simulink model "Problem1"  (R2020b)
settings: Solver=VariableStepAuto  StartTime=0.0  StopTime=120  RelTol=1e-3
model workspace (MAT data in the model file):
  b = Simulink.Parameter
  b.Value = 50
  b.DataType = 'auto'
  b.Dimensions = [1 1]
  m = Simulink.Parameter
  m.Value = 1000
  m.DataType = 'auto'
  m.Dimensions = [1 1]
  u = Simulink.Parameter
  u.Value = 500
  u.DataType = 'auto'
  u.Dimensions = [1 1]
settings Model: Creator=Hp  LastModifiedBy=Hp

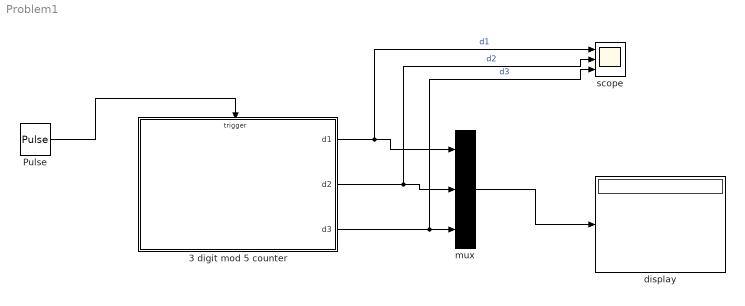
== system Problem1 ==
  3 digit mod 5 counter : Stateflow chart  TreatAsAtomicUnit=on
  Pulse : DiscretePulseGenerator  PulseType=Time based  Period=1  PulseWidth=5
  display : Display
  mux : Mux  Inputs=3
  scope : Scope  NumInputPorts=3
  wires:
  Pulse/1 -> 3 digit mod 5 counter/Trigger
  mux/1 -> display/1
  3 digit mod 5 counter/3(d3) -> scope/3, mux/3  "d3"
  3 digit mod 5 counter/2(d2) -> scope/2, mux/2  "d2"
  3 digit mod 5 counter/1(d1) -> scope/1, mux/1  "d1"

== stateflow chart Problem1/3 digit mod 5 counter ==
  state digit1 [parallel]
    settings: executionOrder=1
    state zero
      en:d1=0;
    state four
      en:d1=4;
    state one
      en:d1=1;
    state three
      en:d1=3;
    state two
      en:d1=2;
    (default) -> digit1.zero
    digit1.zero -> digit1.one : inputClick
    digit1.four -> digit1.zero : inputClick/{digit2.inc2}
    digit1.three -> digit1.four : inputClick
    digit1.one -> digit1.two : inputClick
    digit1.two -> digit1.three : inputClick
  state digit2 [parallel]
    settings: executionOrder=2
    state one
      en:d2=1;
    state zero
      en:d2=0;
    state two
      en:d2=2;
    state four
      en:d2=4;
    state three
      en:d2=3;
    digit2.zero -> digit2.one : inc2
    digit2.one -> digit2.two : inc2
    (default) -> digit2.zero
    digit2.four -> digit2.zero : inc2/{digit3.inc3}
    digit2.two -> digit2.three : inc2
    digit2.three -> digit2.four : inc2
  state digit3 [parallel]
    settings: executionOrder=3
    state two
      en:d3=2;
    state one
      en:d3=1;
    state three
      en:d3=3;
    state zero
      en:d3=0;
    state four
      en:d3=4;
    digit3.one -> digit3.two : inc3
    digit3.two -> digit3.three : inc3
    digit3.zero -> digit3.one : inc3
    digit3.three -> digit3.four : inc3
    digit3.four -> digit3.zero : inc3
    (default) -> digit3.zero
  data: d1 output; d2 output; d3 output
  events: inc2 local FUNCTION_CALL_EVENT; inc3 local FUNCTION_CALL_EVENT; inputClick input RISING_EDGE_EVENT
